simulink model "RST"  (R2022b)
settings: Solver=VariableStepAuto  StartTime=0.0  StopTime=25  RelTol=1e-3
values from neighbouring files (symbols this model uses):
  A = Hd.den{1}    [VariantaBUNA10.m]
  Am = H_0dt.den{1}    [VariantaBUNA10.m]
  B = Hd.num{1}    [VariantaBUNA10.m]
  Bm = H_0dt.num{1}    [VariantaBUNA10.m]
  S = conv(S1, [1, -1])    [VariantaBUNA10.m]
  T = H0d.den{1}/ sum(B)    [VariantaBUNA10.m]
undefined symbols (not defined in the file or in its folder): R
settings Model: Creator=saioc  LastModifiedBy=saioc

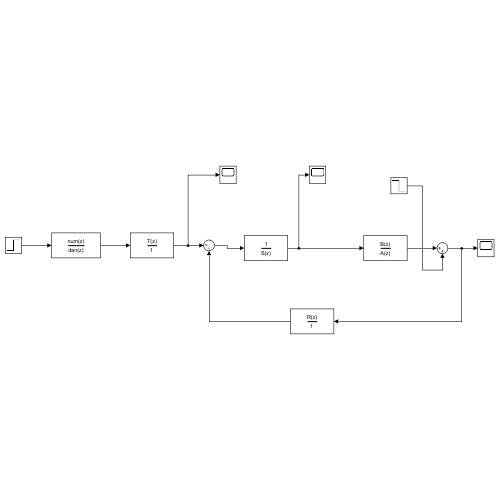
[thumbnail: Simulink's stored preview of the top-level diagram]
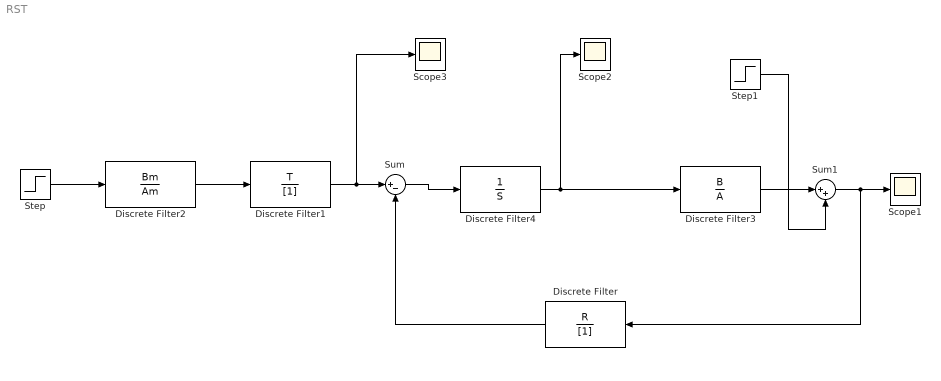
== system RST ==
  Discrete Filter : DiscreteFilter  Numerator=R  Denominator=[1]  SampleTime=0.3
  Discrete Filter1 : DiscreteFilter  Numerator=T  Denominator=[1]  SampleTime=0.3
  Discrete Filter2 : DiscreteFilter  Numerator=Bm  Denominator=Am  SampleTime=0.3
  Discrete Filter3 : DiscreteFilter  Numerator=B  Denominator=A  SampleTime=0.3
  Discrete Filter4 : DiscreteFilter  Numerator=1  Denominator=S  SampleTime=0.3
  Scope1 : Scope
  Scope2 : Scope
  Scope3 : Scope
  Step : Step  After=100  SampleTime=0.3
  Step1 : Step  Time=15  After=-10  SampleTime=0.3
  Sum : Sum  Inputs=|+-
  Sum1 : Sum  Inputs=|++
  wires:
  Sum/1 -> Discrete Filter4/1
  Discrete Filter4/1 -> Discrete Filter3/1, Scope2/1
  Discrete Filter/1 -> Sum/2
  Step/1 -> Discrete Filter2/1
  Discrete Filter1/1 -> Scope3/1, Sum/1
  Discrete Filter2/1 -> Discrete Filter1/1
  Discrete Filter3/1 -> Sum1/1
  Sum1/1 -> Discrete Filter/1, Scope1/1
  Step1/1 -> Sum1/2
